simulink model "tqdtqr_rebuild_V3"  (R2021b)
settings: Solver=VariableStepAuto  StartTime=0.0  StopTime=10.0  RelTol=1e-3
undefined symbols (not defined in the file): ATQD_AfterTqMinGain_X_Deg, ATQD_APSCreepBaseTqD_X_kph, ATQD_APSCreepBaseTqD_Y_Deg, ATQD_APSCreepBaseTqR_X_kph, ATQD_APSCreepBaseTqR_Y_Deg, ATQD_APSCreepIterm_X_kph, ATQD_APSCreepIterm_Y_kph, ATQD_APSCreepPterm_X_kph, ATQD_APSCreepPterm_Y_kph, ATQD_APSDecReq_X_kph, ATQD_APSDecReq_Y_mps2, ATQD_APSDecReqCMD_X_kph, ATQD_APSDecReqTs_X_pct, ATQD_APSDecTimeGain_X_Deg, ATQD_APSDecTimeGain_Y_s, ATQD_APSReqLowSpd_X_Deg, ATQD_AutoHoldReleaseBPS_X_Deg, ATQD_AWDLoadTrqnsGain_X_kg, ATQD_AWDLoadTrqnsGain_Y_pct, ATQD_BOSEnBPSPosn_X_kph, ATQD_BOSMap_X_rpm, ATQD_BOSMap_Y_pct, ATQD_CreepBaseTqD_X_kph, ATQD_CreepBaseTqD_Y_Deg, ATQD_CreepBaseTqR_X_kph, ATQD_CreepBaseTqR_Y_Deg, ATQD_CreepBPSDisPosn_X_Deg, ATQD_CreepBPSDisPosnR_X_Deg, ATQD_CreepBPSEnPosn_X_Deg, ATQD_CreepBPSEnPosnR_X_Deg, ATQD_CreepDeltaTq_X_kph, ATQD_CreepIterm_X_kph, ATQD_CreepIterm_Y_kph, ATQD_CreepItermMaxLimit_X_pct, ATQD_CreepPreloadTime_X_kph, ATQD_CreepPreloadTq_X_kph, ATQD_CreepPreloadTq_Y_s, ATQD_CreepProtTq_X_Deg, ATQD_CreepPterm_X_kph, ATQD_CreepPterm_Y_kph, ATQD_CreepRrTqSpRat_X_rpm, ATQD_CreepRrTqSpRat_Y_Nm, ATQD_CreepTargetSpdD_X_pct, ATQD_CreepTargetSpdR_X_pct, ATQD_CreepUpLimitTq_X_rpm, ATQD_DecIneOPDHoldEnDelay_X_Deg, ATQD_DecIneOPDHoldEnDelay_Y_bar, ATQD_ECOTqMapD_X_rpm, ATQD_ECOTqMapD_Y_pct, ATQD_EMTqMapD_X_rpm, ATQD_EMTqMapD_Y_pct, ATQD_EOPDTqMapDCon_X_rpm, ATQD_EOPDTqMapDCon_Y_Deg, ATQD_EstInitVehWeight_X_c, ATQD_FAfterTqCMDGain_X_rpm, ATQD_FAfterTqCMDGain_Y_pct, ATQD_ForceLowSpd_X_Deg, ATQD_ForcePLimitSpd_X_Deg, ATQD_FrLossMAPLowV_X_rpm, ATQD_FrLossMAPLowV_Y_Nm ... (+949)
libraries: simulink x235, hcu_lib x208, tqr x63, tqd x6
(part 35 of 37)

== stateflow chart tqdtqr_rebuild_V3/Input_Convert/Signal function/SWC1 SWC2 status/SWC2_Subsystem/Speed Setting Mode/ACC Speed Setting ON/ACCSetSpd_2506 ==
  state MeterSpd
    state OFF_Error_Disable
      en:
      VTQD_ACCSetSpd_raw32 =  min(VTQD_ACCActiveMetSpdHi_raw32, VTQD_SpdLim4SetSpd_raw32);
      VTQD_ACCSetSpd_raw32 = max(VTQD_ACCActiveMetSpdLo_raw32, VTQD_ACCSetSpd_raw32);
      VTQD_ACCSavedSetSpd_raw32 = VTQD_ACCSetSpd_raw32;
      du:
      VTQD_ACCSetSpd_raw32 =  min(VTQD_ACCActiveMetSpdHi_raw32, VTQD_SpdLim4SetSpd_raw32);
      VTQD_ACCSetSpd_raw32 = max(VTQD_ACCActiveMetSpdLo_raw32, VTQD_ACCSetSpd_raw32);
      VTQD_ACCSavedSetSpd_raw32 = VTQD_ACCSetSpd_raw32;
    state Terminal
      %Do Nothing
    state Standby
      en:
      VTQD_ACCSetSpd_raw32 =  min(VTQD_ACCActiveMetSpdHi_raw32, VTQD_SpdLim4SetSpd_raw32);
      VTQD_ACCSetSpd_raw32 = max(VTQD_ACCActiveMetSpdLo_raw32, VTQD_ACCSetSpd_raw32);
      VTQD_ACCSavedSetSpd_raw32 = VTQD_ACCSetSpd_raw32;
      du:
      VTQD_ACCSetSpd_raw32 =  min(VTQD_ACCActiveMetSpdHi_raw32, VTQD_SpdLim4SetSpd_raw32);
      VTQD_ACCSetSpd_raw32 = max(VTQD_ACCActiveMetSpdLo_raw32, VTQD_ACCSetSpd_raw32);
      VTQD_ACCSavedSetSpd_raw32 = VTQD_ACCSetSpd_raw32;
    state Active_Override_ShutOff
      (default) -> (junction 749) : {VTQD_HoldResDet_flg = FALSE;
          |  VTQD_ACCSavedSetSpd_raw32 = VTQD_LastSetSpd_kph;
          |  VTQD_ACCSetSpd_raw32 = VTQD_ACCSavedSetSpd_raw32}
      MeterSpd.Active_Override_ShutOff -> (junction 830) [order 1]
      (junction 830) -> (junction 834) [order 1] : [VTQD_DistanceUnit_flg == VINP_Distanceunit_flg || VTQD_ACCSavedSetSpd_raw32 <= ONE_FLOAT]
      (junction 834) -> (junction 749) : {VTQD_ACCSetSpd_raw32 = min(VTQD_ACCActiveMetSpdHi_raw32, VTQD_ACCSavedSetSpd_raw32);
          |  VTQD_ACCSavedSetSpd_raw32 = VTQD_ACCSetSpd_raw32;}
      (junction 749) -> (junction 1142) [order 1] : [VINP_ADASACCSta_enum == ENUM_ADASACCSTA_ACTIVE]
      (junction 1142) -> (junction 1148) [order 1] : [(VTQD_SWC2ScrollUpSta_flg ||...
          |   VTQD_SWC2ScrollDownSta_flg ||...
          |   VTQD_SWC2ScrollUpSta_enum == ENUM_SWCBOTTONPRESS_SHORTPRESS ||...
          |   VTQD_SWC2ScrollDownSta_enum == ENUM_SWCBOTTONPRESS_SHORTPRESS) &&...
          |  VTQD_HoldResDet_flg]
          | %add20250114
      (junction 830) -> (junction 832) [order 2]
      (junction 837) -> (junction 834)
      (junction 749) -> (junction 798) [order 2]
      (junction 1142) -> (junction 1144) [order 2] : {VTQD_HoldResDet_flg = FALSE}
          | %add20250114
      (junction 1148) -> (junction 1146) : {VTQD_HoldResDet_flg = TRUE}
          | %add20250114
      (junction 832) -> (junction 819) [order 1] : [VINP_Distanceunit_flg]
      (junction 832) -> (junction 833) [order 2] : {VTQD_ACCSavedSetSpd_raw32 = (VTQD_ACCSavedSetSpd_raw32 * MPH2KPH)}
      (junction 819) -> (junction 827) : {VTQD_ACCSavedSetSpd_raw32 = (VTQD_ACCSavedSetSpd_raw32 * KPH2MPH)}
      (junction 1144) -> (junction 1146)
      (junction 1146) -> (junction 751)
      (junction 751) -> (junction 757) [order 1] : [VTQD_Set2MeterSpd_flg ||...
          |  VTQD_SetRoadSpdLim_flg]
      (junction 757) -> (junction 1115) [order 1] : [VTQD_Set2MeterSpd_flg]
      (junction 751) -> (junction 762) [order 2]
      (junction 757) -> (junction 759) [order 2] : {VTQD_ACCSetSpd_raw32 =  min(VTQD_ACCActiveMetSpdHi_raw32, VTQD_SpdLim4SetSpd_raw32);
          |  VTQD_ACCSetSpd_raw32 = max(VTQD_ACCActiveMetSpdLo_raw32, VTQD_ACCSetSpd_raw32);
          |  VTQD_ACCSavedSetSpd_raw32 = VTQD_ACCSetSpd_raw32;
          |  VTQD_DistanceUnit_flg = VINP_Distanceunit_flg;}
      (junction 1115) -> (junction 1114) : {VTQD_ACCSetSpd_raw32 =  min(VTQD_ACCActiveMetSpdHi_raw32, VVMC_MeterIndSpeed_raw32);
          |  VTQD_ACCSetSpd_raw32 = max(VTQD_ACCActiveMetSpdLo_raw32, VTQD_ACCSetSpd_raw32);
          |  VTQD_ACCSavedSetSpd_raw32 = VTQD_ACCSetSpd_raw32;
          |  VTQD_DistanceUnit_flg = VINP_Distanceunit_flg;}
      (junction 827) -> (junction 816) [order 1] : [VTQD_ACCSavedSetSpd_raw32 < KTQD_ACCActiveMetSpdLoMPH_mph]
      (junction 833) -> (junction 817) [order 1] : [VTQD_ACCSavedSetSpd_raw32 < KTQD_ACCActiveMetSpdLo_kph]
      (junction 816) -> (junction 820) : {VTQD_ACCSavedSetSpd_raw32 = KTQD_ACCActiveMetSpdLoMPH_mph}
      (junction 833) -> (junction 828) [order 2]
      (junction 817) -> (junction 815) : {VTQD_ACCSavedSetSpd_raw32 = KTQD_ACCActiveMetSpdLo_kph}
      (junction 827) -> (junction 818) [order 2]
      (junction 820) -> (junction 818)
      (junction 815) -> (junction 828)
      (junction 818) -> (junction 826)
      (junction 828) -> (junction 821)
      (junction 762) -> (junction 766) [order 1] : [(VTQD_SWC2ScrollUpSta_enum == ENUM_SWCBOTTONPRESS_SHORTPRESS ||...
          |   VTQD_SWC2ScrollDownSta_enum == ENUM_SWCBOTTONPRESS_SHORTPRESS) &&...
          |  !VVMC_LVDAACCStatusInformation_flg && !VTQD_HoldResDet_flg]
          | %add20250114
      (junction 766) -> (junction 771) [order 1] : [VTQD_SWC2ScrollUpSta_enum == ENUM_SWCBOTTONPRESS_SHORTPRESS]
      (junction 821) -> (junction 829) [order 1] : [VTQD_ACCSavedSetSpd_raw32 > KTQD_ACCActiveMetSpdHi_kph]
      (junction 826) -> (junction 822) [order 1] : [VTQD_ACCSavedSetSpd_raw32 > KTQD_ACCActiveMetSpdHiMPH_mph]
      (junction 762) -> (junction 792) [order 2]
      (junction 766) -> (junction 779) [order 2] : {VTQD_ACCSetSpd_raw32 =  min(VTQD_ACCActiveMetSpdHi_raw32, VTQD_ACCSavedSetSpd_raw32 - ONE_FLOAT);
          |  VTQD_ACCSetSpd_raw32 = max(VTQD_ACCActiveMetSpdLo_raw32, VTQD_ACCSetSpd_raw32);
          |  VTQD_ACCSavedSetSpd_raw32 = VTQD_ACCSetSpd_raw32;
          |  VTQD_DistanceUnit_flg = VINP_Distanceunit_flg;}
      (junction 771) -> (junction 774) : {VTQD_ACCSetSpd_raw32 =  min(VTQD_ACCActiveMetSpdHi_raw32, VTQD_ACCSavedSetSpd_raw32 + ONE_FLOAT);
          |  VTQD_ACCSetSpd_raw32 = max(VTQD_ACCActiveMetSpdLo_raw32, VTQD_ACCSetSpd_raw32);
          |  VTQD_ACCSavedSetSpd_raw32 = VTQD_ACCSetSpd_raw32;
          |  VTQD_DistanceUnit_flg = VINP_Distanceunit_flg;}
      (junction 821) -> (junction 823) [order 2]
      (junction 829) -> (junction 831) : {VTQD_ACCSavedSetSpd_raw32 = KTQD_ACCActiveMetSpdHi_kph}
      (junction 826) -> (junction 835) [order 2]
      (junction 822) -> (junction 824) : {VTQD_ACCSavedSetSpd_raw32 = KTQD_ACCActiveMetSpdHiMPH_mph}
      (junction 831) -> (junction 823)
      (junction 824) -> (junction 835)
      (junction 823) -> (junction 825)
      (junction 835) -> (junction 836)
      (junction 825) -> (junction 836)
      (junction 836) -> (junction 837)
      (junction 792) -> (junction 785) [order 1] : [(VTQD_SWC2ScrollUpSta_enum == ENUM_SWCBOTTONPRESS_LONGPRESS ||...
          |   VTQD_SWC2ScrollDownSta_enum == ENUM_SWCBOTTONPRESS_LONGPRESS) &&...
          |  !VVMC_LVDAACCStatusInformation_flg && !VTQD_HoldResDet_flg]
          | %add20250114
      (junction 785) -> (junction 790) [order 1] : [VTQD_SWC2ScrollUpSta_enum == ENUM_SWCBOTTONPRESS_LONGPRESS]
      (junction 792) -> (junction 1131) [order 2]
      (junction 785) -> (junction 793) [order 2] : {VTQD_ACCSetSpd_raw32 = max(VTQD_ACCActiveMetSpdLo_raw32, ceil(VTQD_ACCSavedSetSpd_raw32 / VTQD_SetSpdDeltaLong_raw32 - ONE_FLOAT) * VTQD_SetSpdDeltaLong_raw32);
          |  VTQD_ACCSetSpd_raw32 = min (VTQD_ACCActiveMetSpdHi_raw32, VTQD_ACCSetSpd_raw32);
          |  VTQD_ACCSavedSetSpd_raw32 = VTQD_ACCSetSpd_raw32;
          |  VTQD_DistanceUnit_flg = VINP_Distanceunit_flg;}
      (junction 790) -> (junction 783) : {VTQD_ACCSetSpd_raw32 = min(VTQD_ACCActiveMetSpdHi_raw32, floor(VTQD_ACCSavedSetSpd_raw32 / VTQD_SetSpdDeltaLong_raw32 + ONE_FLOAT) * VTQD_SetSpdDeltaLong_raw32);
          |  VTQD_ACCSetSpd_raw32 = max (VTQD_ACCActiveMetSpdLo_raw32, VTQD_ACCSetSpd_raw32);
          |  VTQD_ACCSavedSetSpd_raw32 = VTQD_ACCSetSpd_raw32;
          |  VTQD_DistanceUnit_flg = VINP_Distanceunit_flg;}
      (junction 1131) -> (junction 1133) [order 1] : [(VTQD_SWC2ScrollUpSta_flg ||...
          |   VTQD_SWC2ScrollDownSta_flg) &&...
          |  VVMC_LVDAACCStatusInformation_flg]
          | %add20250114
      (junction 1131) -> (junction 1137) [order 2]
      (junction 1133) -> (junction 1134) : {VTQD_HoldResDet_flg = TRUE}
          | %add20250114
      (junction 1134) -> (junction 1137)
      (junction 1137) -> (junction 1265) : {VTQD_ACCSetSpd_raw32 = VTQD_ACCSavedSetSpd_raw32;
          |  VTQD_ACCSavedSetSpd_raw32 = VTQD_ACCSetSpd_raw32;
          |  VTQD_DistanceUnit_flg = VINP_Distanceunit_flg;}
      (junction 798) -> (junction 1240) [order 1] : [VINP_ADASACCSta_enum == ENUM_ADASACCSTA_OVERRIDE]
      (junction 1240) -> (junction 1235) [order 1] : [KTQD_ACCOVRDSpdAdj_flg &&...
          | (VTQD_Set2MeterSpd_flg ||...
          |  VTQD_SetRoadSpdLim_flg)]
      (junction 1235) -> (junction 1247) [order 1] : [VTQD_Set2MeterSpd_flg]
      (junction 798) -> (junction 807) [order 2] : {VTQD_ACCSetSpd_raw32 = VTQD_ACCSavedSetSpd_raw32;
          |  VTQD_ACCSavedSetSpd_raw32 = VTQD_ACCSetSpd_raw32;
          |  VTQD_DistanceUnit_flg = VINP_Distanceunit_flg;}
      (junction 1240) -> (junction 1236) [order 2]
      (junction 1235) -> (junction 1244) [order 2] : {VTQD_ACCSetSpd_raw32 =  min(VTQD_ACCActiveMetSpdHi_raw32, VTQD_SpdLim4SetSpd_raw32);
          |  VTQD_ACCSetSpd_raw32 = max(VTQD_ACCActiveMetSpdLo_raw32, VTQD_ACCSetSpd_raw32);
          |  VTQD_ACCSavedSetSpd_raw32 = VTQD_ACCSetSpd_raw32;
          |  VTQD_DistanceUnit_flg = VINP_Distanceunit_flg;}
      (junction 1247) -> (junction 1241) : {VTQD_ACCSetSpd_raw32 =  min(VTQD_ACCActiveMetSpdHi_raw32, VVMC_MeterIndSpeed_raw32);
          |  VTQD_ACCSetSpd_raw32 = max(VTQD_ACCActiveMetSpdLo_raw32, VTQD_ACCSetSpd_raw32);
          |  VTQD_ACCSavedSetSpd_raw32 = VTQD_ACCSetSpd_raw32;
          |  VTQD_DistanceUnit_flg = VINP_Distanceunit_flg;}
      (junction 1236) -> (junction 1242) [order 1] : [(VTQD_SWC2ScrollUpSta_enum == ENUM_SWCBOTTONPRESS_SHORTPRESS ||...
          |   VTQD_SWC2ScrollDownSta_enum == ENUM_SWCBOTTONPRESS_SHORTPRESS)]
      (junction 1242) -> (junction 1238) [order 1] : [VTQD_SWC2ScrollUpSta_enum == ENUM_SWCBOTTONPRESS_SHORTPRESS]
      (junction 1236) -> (junction 1245) [order 2]
      (junction 1242) -> (junction 1248) [order 2] : {VTQD_ACCSetSpd_raw32 =  min(VTQD_ACCActiveMetSpdHi_raw32, VTQD_ACCSavedSetSpd_raw32 - ONE_FLOAT);
          |  VTQD_ACCSetSpd_raw32 = max(VTQD_ACCActiveMetSpdLo_raw32, VTQD_ACCSetSpd_raw32);
          |  VTQD_ACCSavedSetSpd_raw32 = VTQD_ACCSetSpd_raw32;
          |  VTQD_DistanceUnit_flg = VINP_Distanceunit_flg;}
      (junction 1238) -> (junction 1239) : {VTQD_ACCSetSpd_raw32 =  min(VTQD_ACCActiveMetSpdHi_raw32, VTQD_ACCSavedSetSpd_raw32 + ONE_FLOAT);
          |  VTQD_ACCSetSpd_raw32 = max(VTQD_ACCActiveMetSpdLo_raw32, VTQD_ACCSetSpd_raw32);
          |  VTQD_ACCSavedSetSpd_raw32 = VTQD_ACCSetSpd_raw32;
          |  VTQD_DistanceUnit_flg = VINP_Distanceunit_flg;}
      (junction 1245) -> (junction 1249) [order 1] : [(VTQD_SWC2ScrollUpSta_enum == ENUM_SWCBOTTONPRESS_LONGPRESS ||...
          |   VTQD_SWC2ScrollDownSta_enum == ENUM_SWCBOTTONPRESS_LONGPRESS)]
      (junction 1249) -> (junction 1243) [order 1] : [VTQD_SWC2ScrollUpSta_enum == ENUM_SWCBOTTONPRESS_LONGPRESS]
      (junction 1245) -> (junction 1234) [order 2] : {VTQD_ACCSetSpd_raw32 = VTQD_ACCSavedSetSpd_raw32;
          |  VTQD_ACCSavedSetSpd_raw32 = VTQD_ACCSetSpd_raw32;
          |  VTQD_DistanceUnit_flg = VINP_Distanceunit_flg;}
      (junction 1249) -> (junction 1246) [order 2] : {VTQD_ACCSetSpd_raw32 = max(VTQD_ACCActiveMetSpdLo_raw32, ceil(VTQD_ACCSavedSetSpd_raw32 / VTQD_SetSpdDeltaLong_raw32 - ONE_FLOAT) * VTQD_SetSpdDeltaLong_raw32);
          |  VTQD_ACCSetSpd_raw32 = min (VTQD_ACCActiveMetSpdHi_raw32, VTQD_ACCSetSpd_raw32);
          |  VTQD_ACCSavedSetSpd_raw32 = VTQD_ACCSetSpd_raw32;
          |  VTQD_DistanceUnit_flg = VINP_Distanceunit_flg;}
      (junction 1243) -> (junction 1237) : {VTQD_ACCSetSpd_raw32 = min(VTQD_ACCActiveMetSpdHi_raw32, floor(VTQD_ACCSavedSetSpd_raw32 / VTQD_SetSpdDeltaLong_raw32 + ONE_FLOAT) * VTQD_SetSpdDeltaLong_raw32);
          |  VTQD_ACCSetSpd_raw32 = max (VTQD_ACCActiveMetSpdLo_raw32, VTQD_ACCSetSpd_raw32);
          |  VTQD_ACCSavedSetSpd_raw32 = VTQD_ACCSetSpd_raw32;
          |  VTQD_DistanceUnit_flg = VINP_Distanceunit_flg;}
    (default) -> MeterSpd.OFF_Error_Disable [order 3]
    MeterSpd.Terminal -> MeterSpd.OFF_Error_Disable [order 2] : [VINP_ADASACCSta_enum ~= ENUM_ADASACCSTA_ACTIVE &&...
        |  VINP_ADASACCSta_enum ~= ENUM_ADASACCSTA_OVERRIDE &&...
        |  VINP_ADASACCSta_enum ~= ENUM_ADASACCSTA_SHUTOFF]
    MeterSpd.OFF_Error_Disable -> MeterSpd.Terminal [order 2] : [VINP_ADASACCSta_enum == ENUM_ADASACCSTA_ACTIVE ||...
        |  VINP_ADASACCSta_enum == ENUM_ADASACCSTA_OVERRIDE ||...
        |  VINP_ADASACCSta_enum == ENUM_ADASACCSTA_SHUTOFF]
    MeterSpd.Terminal -> MeterSpd.Active_Override_ShutOff [order 1] : [VINP_ADASACCSta_enum == ENUM_ADASACCSTA_ACTIVE ||...
        |  VINP_ADASACCSta_enum == ENUM_ADASACCSTA_OVERRIDE ||...
        |  VINP_ADASACCSta_enum == ENUM_ADASACCSTA_SHUTOFF]
    MeterSpd.Active_Override_ShutOff -> MeterSpd.Terminal [order 2] : [VINP_ADASACCSta_enum ~= ENUM_ADASACCSTA_ACTIVE &&...
        |  VINP_ADASACCSta_enum ~= ENUM_ADASACCSTA_OVERRIDE &&...
        |  VINP_ADASACCSta_enum ~= ENUM_ADASACCSTA_SHUTOFF]
    MeterSpd.OFF_Error_Disable -> MeterSpd.Standby [order 1] : [VINP_ADASACCSta_enum == ENUM_ADASACCSTA_STANDBY]
    MeterSpd.Standby -> MeterSpd.OFF_Error_Disable [order 2] : [VINP_ADASACCSta_enum ~= ENUM_ADASACCSTA_STANDBY]
    MeterSpd.Active_Override_ShutOff -> MeterSpd.Standby [order 1] : [VINP_ADASACCSta_enum == ENUM_ADASACCSTA_STANDBY]
    MeterSpd.Standby -> MeterSpd.Active_Override_ShutOff [order 1] : [VINP_ADASACCSta_enum == ENUM_ADASACCSTA_ACTIVE ||...
        |  VINP_ADASACCSta_enum == ENUM_ADASACCSTA_OVERRIDE ||...
        |  VINP_ADASACCSta_enum == ENUM_ADASACCSTA_SHUTOFF]
    (default) -> MeterSpd.Active_Override_ShutOff [order 2] : [VINP_ADASACCSta_enum == ENUM_ADASACCSTA_ACTIVE ||...
        |  VINP_ADASACCSta_enum == ENUM_ADASACCSTA_OVERRIDE ||...
        |  VINP_ADASACCSta_enum == ENUM_ADASACCSTA_SHUTOFF]
    (default) -> MeterSpd.Standby [order 1] : [VINP_ADASACCSta_enum == ENUM_ADASACCSTA_STANDBY]
  state RoadSpd
    state OFF_Error_Disable
      en:
      VTQD_ACCSetSpd_raw32 =  min(VTQD_ACCActiveMetSpdHi_raw32, VTQD_SpdLim4SetSpd_raw32);
      VTQD_ACCSetSpd_raw32 = max(VTQD_ACCActiveMetSpdLo_raw32, VTQD_ACCSetSpd_raw32);
      VTQD_ACCSavedSetSpd_raw32 = VTQD_ACCSetSpd_raw32;
      du:
      VTQD_ACCSetSpd_raw32 =  min(VTQD_ACCActiveMetSpdHi_raw32, VTQD_SpdLim4SetSpd_raw32);
      VTQD_ACCSetSpd_raw32 = max(VTQD_ACCActiveMetSpdLo_raw32, VTQD_ACCSetSpd_raw32);
      VTQD_ACCSavedSetSpd_raw32 = VTQD_ACCSetSpd_raw32;
    state Terminal
      %Do Nothing
    state Standby
      (default) -> (junction 987) : {VTQD_StandbyDisRoadSpd_flg = FALSE;}
      RoadSpd.Standby -> (junction 1029) [order 1]
      (junction 1029) -> (junction 1030) [order 1] : [VTQD_DistanceUnit_flg == VINP_Distanceunit_flg || VTQD_ACCSavedSetSpd_raw32 <= ONE_FLOAT]
      (junction 1030) -> (junction 987) : {VTQD_ACCSetSpd_raw32 = min(VTQD_ACCActiveMetSpdHi_raw32, VTQD_ACCSavedSetSpd_raw32);
          |  VTQD_ACCSavedSetSpd_raw32 = VTQD_ACCSetSpd_raw32;}
      (junction 987) -> (junction 1102) [order 1] : [VTQD_RoadSpdActive2Standby_flg &&...
          | (VTQD_StandbyDisRoadSpd_flg || !VTQD_ADASSLIFSpdLimDet_flg)]
      (junction 1029) -> (junction 1031) [order 2]
      (junction 1048) -> (junction 1030)
      (junction 987) -> (junction 1104) [order 2]
      (junction 1102) -> (junction 999)
      (junction 1031) -> (junction 1032) [order 1] : [VINP_Distanceunit_flg]
      (junction 1031) -> (junction 1034) [order 2] : {VTQD_ACCSavedSetSpd_raw32 = (VTQD_ACCSavedSetSpd_raw32 * MPH2KPH)}
      (junction 1032) -> (junction 1028) : {VTQD_ACCSavedSetSpd_raw32 = (VTQD_ACCSavedSetSpd_raw32 * KPH2MPH)}
      (junction 1104) -> (junction 999) [order 1] : [VTQD_SWC2ScrollUpSta_enum ~= ENUM_SWCBOTTONPRESS_NOPRESS ||...
          |  VTQD_SWC2ScrollDownSta_enum ~= ENUM_SWCBOTTONPRESS_NOPRESS ||...
          |  VTQD_StandbyDisRoadSpd_flg]
      (junction 999) -> (junction 1000) [order 1] : [VTQD_SWC2ScrollUpSta_enum == ENUM_SWCBOTTONPRESS_SHORTPRESS ||...
          |  VTQD_SWC2ScrollDownSta_enum == ENUM_SWCBOTTONPRESS_SHORTPRESS]
      (junction 1000) -> (junction 1001) [order 1] : [VTQD_SWC2ScrollUpSta_enum == ENUM_SWCBOTTONPRESS_SHORTPRESS]
      (junction 1104) -> (junction 991) [order 2] : {VTQD_ACCSetSpd_raw32 =  min(VTQD_ACCActiveMetSpdHi_raw32, VTQD_SpdLim4SetSpd_raw32);
          |  VTQD_ACCSetSpd_raw32 = max(VTQD_ACCActiveMetSpdLo_raw32, VTQD_ACCSetSpd_raw32);
          |  VTQD_ACCSavedSetSpd_raw32 = VTQD_ACCSetSpd_raw32;
          |  VTQD_DistanceUnit_flg = VINP_Distanceunit_flg;
          |  VTQD_RoadSpdActive2Standby_flg = FALSE;}
      (junction 999) -> (junction 1007) [order 2]
      (junction 1000) -> (junction 1005) [order 2] : {VTQD_ACCSetSpd_raw32 =  min(VTQD_ACCActiveMetSpdHi_raw32, VTQD_ACCSavedSetSpd_raw32 - ONE_FLOAT);
          |  VTQD_ACCSetSpd_raw32 = max(VTQD_ACCActiveMetSpdLo_raw32, VTQD_ACCSetSpd_raw32);
          |  VTQD_ACCSavedSetSpd_raw32 = VTQD_ACCSetSpd_raw32;
          |  VTQD_DistanceUnit_flg = VINP_Distanceunit_flg;
          |  VTQD_StandbyDisRoadSpd_flg = TRUE;}
      (junction 1001) -> (junction 1006) : {VTQD_ACCSetSpd_raw32 =  min(VTQD_ACCActiveMetSpdHi_raw32, VTQD_ACCSavedSetSpd_raw32 + ONE_FLOAT);
          |  VTQD_ACCSetSpd_raw32 = max(VTQD_ACCActiveMetSpdLo_raw32, VTQD_ACCSetSpd_raw32);
          |  VTQD_ACCSavedSetSpd_raw32 = VTQD_ACCSetSpd_raw32;
          |  VTQD_DistanceUnit_flg = VINP_Distanceunit_flg;
          |  VTQD_StandbyDisRoadSpd_flg = TRUE;}
      (junction 1028) -> (junction 1033) [order 1] : [VTQD_ACCSavedSetSpd_raw32 < KTQD_ACCActiveMetSpdLoMPH_mph]
      (junction 1034) -> (junction 1035) [order 1] : [VTQD_ACCSavedSetSpd_raw32 < KTQD_ACCActiveMetSpdLo_kph]
      (junction 1033) -> (junction 1043) : {VTQD_ACCSavedSetSpd_raw32 = KTQD_ACCActiveMetSpdLoMPH_mph}
      (junction 1034) -> (junction 1038) [order 2]
      (junction 1035) -> (junction 1039) : {VTQD_ACCSavedSetSpd_raw32 = KTQD_ACCActiveMetSpdLo_kph}
      (junction 1028) -> (junction 1045) [order 2]
      (junction 1043) -> (junction 1045)
      (junction 1039) -> (junction 1038)
      (junction 1045) -> (junction 1042)
      (junction 1038) -> (junction 1040)
      (junction 1040) -> (junction 1041) [order 1] : [VTQD_ACCSavedSetSpd_raw32 > KTQD_ACCActiveMetSpdHi_kph]
      (junction 1042) -> (junction 1044) [order 1] : [VTQD_ACCSavedSetSpd_raw32 > KTQD_ACCActiveMetSpdHiMPH_mph]
      (junction 1040) -> (junction 1053) [order 2]
      (junction 1041) -> (junction 1049) : {VTQD_ACCSavedSetSpd_raw32 = KTQD_ACCActiveMetSpdHi_kph}
      (junction 1042) -> (junction 1054) [order 2]
      (junction 1044) -> (junction 1047) : {VTQD_ACCSavedSetSpd_raw32 = KTQD_ACCActiveMetSpdHiMPH_mph}
      (junction 1007) -> (junction 1011) [order 1] : [VTQD_SWC2ScrollUpSta_enum == ENUM_SWCBOTTONPRESS_LONGPRESS ||...
          |  VTQD_SWC2ScrollDownSta_enum == ENUM_SWCBOTTONPRESS_LONGPRESS]
      (junction 1011) -> (junction 1009) [order 1] : [VTQD_SWC2ScrollUpSta_enum == ENUM_SWCBOTTONPRESS_LONGPRESS]
      (junction 1007) -> (junction 1012) [order 2]
      (junction 1011) -> (junction 1010) [order 2] : {VTQD_ACCSetSpd_raw32 = max(VTQD_ACCActiveMetSpdLo_raw32, ceil(VTQD_ACCSavedSetSpd_raw32 / VTQD_SetSpdDeltaLong_raw32 - ONE_FLOAT) * VTQD_SetSpdDeltaLong_raw32);
          |  VTQD_ACCSetSpd_raw32 = min (VTQD_ACCActiveMetSpdHi_raw32, VTQD_ACCSetSpd_raw32);
          |  VTQD_ACCSavedSetSpd_raw32 = VTQD_ACCSetSpd_raw32;
          |  VTQD_DistanceUnit_flg = VINP_Distanceunit_flg;
          |  VTQD_StandbyDisRoadSpd_flg = TRUE;}
      (junction 1009) -> (junction 1008) : {VTQD_ACCSetSpd_raw32 = min(VTQD_ACCActiveMetSpdHi_raw32, floor(VTQD_ACCSavedSetSpd_raw32 / VTQD_SetSpdDeltaLong_raw32 + ONE_FLOAT) * VTQD_SetSpdDeltaLong_raw32);
          |  VTQD_ACCSetSpd_raw32 = max (VTQD_ACCActiveMetSpdLo_raw32, VTQD_ACCSetSpd_raw32);
          |  VTQD_ACCSavedSetSpd_raw32 = VTQD_ACCSetSpd_raw32;
          |  VTQD_DistanceUnit_flg = VINP_Distanceunit_flg;
          |  VTQD_StandbyDisRoadSpd_flg = TRUE;}
      (junction 1049) -> (junction 1053)
      (junction 1047) -> (junction 1054)
      (junction 1053) -> (junction 1046)
      (junction 1054) -> (junction 1050)
      (junction 1046) -> (junction 1050)
      (junction 1050) -> (junction 1048)
      (junction 1012) -> (junction 1023) [order 1] : [VTQD_LScrollPressShort_flg &&...
          |  VTQD_ADASSLIFSpdLimDet_flg]
      (junction 1023) -> (junction 1026) : {VTQD_ACCSetSpd_raw32 =  min(VTQD_ACCActiveMetSpdHi_raw32, VTQD_SpdLim4SetSpd_raw32);
          |  VTQD_ACCSetSpd_raw32 = max(VTQD_ACCActiveMetSpdLo_raw32, VTQD_ACCSetSpd_raw32);
          |  VTQD_ACCSavedSetSpd_raw32 = VTQD_ACCSetSpd_raw32;
          |  VTQD_DistanceUnit_flg = VINP_Distanceunit_flg;
          |  VTQD_StandbyDisRoadSpd_flg = FALSE;
          |  VTQD_RoadSpdActive2Standby_flg = FALSE;}
      (junction 1012) -> (junction 1022) [order 2] : {VTQD_ACCSetSpd_raw32 =  VTQD_ACCSavedSetSpd_raw32;
          |  VTQD_ACCSavedSetSpd_raw32 = VTQD_ACCSetSpd_raw32;
          |  VTQD_DistanceUnit_flg = VINP_Distanceunit_flg;}
    state Active_Override_ShutOff
      (default) -> (junction 883) : {VTQD_HoldResDet_flg = FALSE;
          |  VTQD_ACCSavedSetSpd_raw32 = VTQD_LastSetSpd_kph;
          |  VTQD_ACCSetSpd_raw32 = VTQD_ACCSavedSetSpd_raw32}
      RoadSpd.Active_Override_ShutOff -> (junction 881) [order 1]
      (junction 881) -> (junction 882) [order 1] : [VTQD_DistanceUnit_flg == VINP_Distanceunit_flg || VTQD_ACCSavedSetSpd_raw32 <= ONE_FLOAT]
      (junction 882) -> (junction 883) : {VTQD_ACCSetSpd_raw32 = min(VTQD_ACCActiveMetSpdHi_raw32, VTQD_ACCSavedSetSpd_raw32);
          |  VTQD_ACCSavedSetSpd_raw32 = VTQD_ACCSetSpd_raw32;}
      (junction 883) -> (junction 1190) [order 1] : [VINP_ADASACCSta_enum == ENUM_ADASACCSTA_ACTIVE]
      (junction 1190) -> (junction 1197) [order 1] : [(VTQD_SWC2ScrollUpSta_flg ||...
          |   VTQD_SWC2ScrollDownSta_flg ||...
          |   VTQD_SWC2ScrollUpSta_enum == ENUM_SWCBOTTONPRESS_SHORTPRESS ||...
          |   VTQD_SWC2ScrollDownSta_enum == ENUM_SWCBOTTONPRESS_SHORTPRESS) &&...
          |  VTQD_HoldResDet_flg]
          | %add20250114
      (junction 881) -> (junction 886) [order 2]
      (junction 915) -> (junction 882)
      (junction 883) -> (junction 919) [order 2]
      (junction 1190) -> (junction 1193) [order 2] : {VTQD_HoldResDet_flg = FALSE}
          | %add20250114
      (junction 1197) -> (junction 1195) : {VTQD_HoldResDet_flg = TRUE}
          | %add20250114
      (junction 886) -> (junction 887) [order 1] : [VINP_Distanceunit_flg]
      (junction 886) -> (junction 893) [order 2] : {VTQD_ACCSavedSetSpd_raw32 = (VTQD_ACCSavedSetSpd_raw32 * MPH2KPH)}
      (junction 887) -> (junction 895) : {VTQD_ACCSavedSetSpd_raw32 = (VTQD_ACCSavedSetSpd_raw32 * KPH2MPH)}
      (junction 1193) -> (junction 1195)
      (junction 1195) -> (junction 884)
      (junction 884) -> (junction 885) [order 1] : [VTQD_Set2MeterSpd_flg ||...
          |  VTQD_SetRoadSpdLim_flg]
      (junction 885) -> (junction 1124) [order 1] : [VTQD_Set2MeterSpd_flg]
      (junction 884) -> (junction 889) [order 2]
      (junction 885) -> (junction 888) [order 2] : {VTQD_ACCSetSpd_raw32 =  min(VTQD_ACCActiveMetSpdHi_raw32, VTQD_SpdLim4SetSpd_raw32);
          |  VTQD_ACCSetSpd_raw32 = max(VTQD_ACCActiveMetSpdLo_raw32, VTQD_ACCSetSpd_raw32);
          |  VTQD_ACCSavedSetSpd_raw32 = VTQD_ACCSetSpd_raw32;
          |  VTQD_DistanceUnit_flg = VINP_Distanceunit_flg;}
      (junction 1124) -> (junction 1123) : {VTQD_ACCSetSpd_raw32 =  min(VTQD_ACCActiveMetSpdHi_raw32, VVMC_MeterIndSpeed_raw32);
          |  VTQD_ACCSetSpd_raw32 = max(VTQD_ACCActiveMetSpdLo_raw32, VTQD_ACCSetSpd_raw32);
          |  VTQD_ACCSavedSetSpd_raw32 = VTQD_ACCSetSpd_raw32;
          |  VTQD_DistanceUnit_flg = VINP_Distanceunit_flg;}
      (junction 895) -> (junction 892) [order 1] : [VTQD_ACCSavedSetSpd_raw32 < KTQD_ACCActiveMetSpdLoMPH_mph]
      (junction 893) -> (junction 894) [order 1] : [VTQD_ACCSavedSetSpd_raw32 < KTQD_ACCActiveMetSpdLo_kph]
      (junction 892) -> (junction 897) : {VTQD_ACCSavedSetSpd_raw32 = KTQD_ACCActiveMetSpdLoMPH_mph}
      (junction 893) -> (junction 898) [order 2]
      (junction 894) -> (junction 899) : {VTQD_ACCSavedSetSpd_raw32 = KTQD_ACCActiveMetSpdLo_kph}
      (junction 895) -> (junction 896) [order 2]
      (junction 897) -> (junction 896)
      (junction 899) -> (junction 898)
      (junction 896) -> (junction 902)
      (junction 898) -> (junction 900)
      (junction 889) -> (junction 890) [order 1] : [(VTQD_SWC2ScrollUpSta_enum == ENUM_SWCBOTTONPRESS_SHORTPRESS ||...
          |   VTQD_SWC2ScrollDownSta_enum == ENUM_SWCBOTTONPRESS_SHORTPRESS) &&...
          |  !VVMC_LVDAACCStatusInformation_flg && !VTQD_HoldResDet_flg]
          | %add20250114
      (junction 890) -> (junction 891) [order 1] : [VTQD_SWC2ScrollUpSta_enum == ENUM_SWCBOTTONPRESS_SHORTPRESS]
      (junction 900) -> (junction 901) [order 1] : [VTQD_ACCSavedSetSpd_raw32 > KTQD_ACCActiveMetSpdHi_kph]
      (junction 902) -> (junction 903) [order 1] : [VTQD_ACCSavedSetSpd_raw32 > KTQD_ACCActiveMetSpdHiMPH_mph]
      (junction 889) -> (junction 906) [order 2]
      (junction 890) -> (junction 904) [order 2] : {VTQD_ACCSetSpd_raw32 =  min(VTQD_ACCActiveMetSpdHi_raw32, VTQD_ACCSavedSetSpd_raw32 - ONE_FLOAT);
          |  VTQD_ACCSetSpd_raw32 = max(VTQD_ACCActiveMetSpdLo_raw32, VTQD_ACCSetSpd_raw32);
          |  VTQD_ACCSavedSetSpd_raw32 = VTQD_ACCSetSpd_raw32;
          |  VTQD_DistanceUnit_flg = VINP_Distanceunit_flg;}
      (junction 891) -> (junction 905) : {VTQD_ACCSetSpd_raw32 =  min(VTQD_ACCActiveMetSpdHi_raw32, VTQD_ACCSavedSetSpd_raw32 + ONE_FLOAT);
          |  VTQD_ACCSetSpd_raw32 = max(VTQD_ACCActiveMetSpdLo_raw32, VTQD_ACCSetSpd_raw32);
          |  VTQD_ACCSavedSetSpd_raw32 = VTQD_ACCSetSpd_raw32;
          |  VTQD_DistanceUnit_flg = VINP_Distanceunit_flg;}
      (junction 900) -> (junction 909) [order 2]
      (junction 901) -> (junction 910) : {VTQD_ACCSavedSetSpd_raw32 = KTQD_ACCActiveMetSpdHi_kph}
      (junction 902) -> (junction 911) [order 2]
      (junction 903) -> (junction 912) : {VTQD_ACCSavedSetSpd_raw32 = KTQD_ACCActiveMetSpdHiMPH_mph}
      (junction 910) -> (junction 909)
      (junction 912) -> (junction 911)
      (junction 909) -> (junction 913)
      (junction 911) -> (junction 914)
      (junction 913) -> (junction 914)
      (junction 914) -> (junction 915)
      (junction 906) -> (junction 907) [order 1] : [(VTQD_SWC2ScrollUpSta_enum == ENUM_SWCBOTTONPRESS_LONGPRESS ||...
          |   VTQD_SWC2ScrollDownSta_enum == ENUM_SWCBOTTONPRESS_LONGPRESS) &&...
          |  !VVMC_LVDAACCStatusInformation_flg && !VTQD_HoldResDet_flg]
          | %add20250114
      (junction 907) -> (junction 908) [order 1] : [VTQD_SWC2ScrollUpSta_enum == ENUM_SWCBOTTONPRESS_LONGPRESS]
      (junction 906) -> (junction 1200) [order 2]
      (junction 907) -> (junction 917) [order 2] : {VTQD_ACCSetSpd_raw32 = max(VTQD_ACCActiveMetSpdLo_raw32, ceil(VTQD_ACCSavedSetSpd_raw32 / VTQD_SetSpdDeltaLong_raw32 - ONE_FLOAT) * VTQD_SetSpdDeltaLong_raw32);
          |  VTQD_ACCSetSpd_raw32 = min (VTQD_ACCActiveMetSpdHi_raw32, VTQD_ACCSetSpd_raw32);
          |  VTQD_ACCSavedSetSpd_raw32 = VTQD_ACCSetSpd_raw32;
          |  VTQD_DistanceUnit_flg = VINP_Distanceunit_flg;}
      (junction 908) -> (junction 918) : {VTQD_ACCSetSpd_raw32 = min(VTQD_ACCActiveMetSpdHi_raw32, floor(VTQD_ACCSavedSetSpd_raw32 / VTQD_SetSpdDeltaLong_raw32 + ONE_FLOAT) * VTQD_SetSpdDeltaLong_raw32);
          |  VTQD_ACCSetSpd_raw32 = max (VTQD_ACCActiveMetSpdLo_raw32, VTQD_ACCSetSpd_raw32);
          |  VTQD_ACCSavedSetSpd_raw32 = VTQD_ACCSetSpd_raw32;
          |  VTQD_DistanceUnit_flg = VINP_Distanceunit_flg;}
      (junction 1200) -> (junction 1209) [order 1] : [(VTQD_SWC2ScrollUpSta_flg ||...
          |   VTQD_SWC2ScrollDownSta_flg) &&...
          |  VVMC_LVDAACCStatusInformation_flg]
          | %add20250114
      (junction 1200) -> (junction 1202) [order 2]
      (junction 1209) -> (junction 1207) : {VTQD_HoldResDet_flg = TRUE}
          | %add20250114
      (junction 1207) -> (junction 1202)
      (junction 1202) -> (junction 1204) : {VTQD_ACCSetSpd_raw32 = VTQD_ACCSavedSetSpd_raw32;
          |  VTQD_ACCSavedSetSpd_raw32 = VTQD_ACCSetSpd_raw32;
          |  VTQD_DistanceUnit_flg = VINP_Distanceunit_flg;}
      (junction 919) -> (junction 1278) [order 1] : [VINP_ADASACCSta_enum == ENUM_ADASACCSTA_OVERRIDE]
      (junction 1278) -> (junction 1266) [order 1] : [KTQD_ACCOVRDSpdAdj_flg &&...
          | (VTQD_Set2MeterSpd_flg ||...
          |  VTQD_SetRoadSpdLim_flg)]
      (junction 1266) -> (junction 1277) [order 1] : [VTQD_Set2MeterSpd_flg]
      (junction 919) -> (junction 924) [order 2] : {VTQD_ACCSetSpd_raw32 = VTQD_ACCSavedSetSpd_raw32;
          |  VTQD_ACCSavedSetSpd_raw32 = VTQD_ACCSetSpd_raw32;
          |  VTQD_DistanceUnit_flg = VINP_Distanceunit_flg;}
      (junction 1278) -> (junction 1268) [order 2]
      (junction 1266) -> (junction 1272) [order 2] : {VTQD_ACCSetSpd_raw32 =  min(VTQD_ACCActiveMetSpdHi_raw32, VTQD_SpdLim4SetSpd_raw32);
          |  VTQD_ACCSetSpd_raw32 = max(VTQD_ACCActiveMetSpdLo_raw32, VTQD_ACCSetSpd_raw32);
          |  VTQD_ACCSavedSetSpd_raw32 = VTQD_ACCSetSpd_raw32;
          |  VTQD_DistanceUnit_flg = VINP_Distanceunit_flg;}
      (junction 1277) -> (junction 1269) : {VTQD_ACCSetSpd_raw32 =  min(VTQD_ACCActiveMetSpdHi_raw32, VVMC_MeterIndSpeed_raw32);
          |  VTQD_ACCSetSpd_raw32 = max(VTQD_ACCActiveMetSpdLo_raw32, VTQD_ACCSetSpd_raw32);
          |  VTQD_ACCSavedSetSpd_raw32 = VTQD_ACCSetSpd_raw32;
          |  VTQD_DistanceUnit_flg = VINP_Distanceunit_flg;}
      (junction 1268) -> (junction 1280) [order 1] : [(VTQD_SWC2ScrollUpSta_enum == ENUM_SWCBOTTONPRESS_SHORTPRESS ||...
          |   VTQD_SWC2ScrollDownSta_enum == ENUM_SWCBOTTONPRESS_SHORTPRESS)]
      (junction 1280) -> (junction 1270) [order 1] : [VTQD_SWC2ScrollUpSta_enum == ENUM_SWCBOTTONPRESS_SHORTPRESS]
      (junction 1268) -> (junction 1276) [order 2]
      (junction 1280) -> (junction 1279) [order 2] : {VTQD_ACCSetSpd_raw32 =  min(VTQD_ACCActiveMetSpdHi_raw32, VTQD_ACCSavedSetSpd_raw32 - ONE_FLOAT);
          |  VTQD_ACCSetSpd_raw32 = max(VTQD_ACCActiveMetSpdLo_raw32, VTQD_ACCSetSpd_raw32);
          |  VTQD_ACCSavedSetSpd_raw32 = VTQD_ACCSetSpd_raw32;
          |  VTQD_DistanceUnit_flg = VINP_Distanceunit_flg;}
      (junction 1270) -> (junction 1274) : {VTQD_ACCSetSpd_raw32 =  min(VTQD_ACCActiveMetSpdHi_raw32, VTQD_ACCSavedSetSpd_raw32 + ONE_FLOAT);
          |  VTQD_ACCSetSpd_raw32 = max(VTQD_ACCActiveMetSpdLo_raw32, VTQD_ACCSetSpd_raw32);
          |  VTQD_ACCSavedSetSpd_raw32 = VTQD_ACCSetSpd_raw32;
          |  VTQD_DistanceUnit_flg = VINP_Distanceunit_flg;}
      (junction 1276) -> (junction 1285) [order 1] : [(VTQD_SWC2ScrollUpSta_enum == ENUM_SWCBOTTONPRESS_LONGPRESS ||...
          |   VTQD_SWC2ScrollDownSta_enum == ENUM_SWCBOTTONPRESS_LONGPRESS)]
      (junction 1285) -> (junction 1271) [order 1] : [VTQD_SWC2ScrollUpSta_enum == ENUM_SWCBOTTONPRESS_LONGPRESS]
      (junction 1276) -> (junction 1267) [order 2] : {VTQD_ACCSetSpd_raw32 = VTQD_ACCSavedSetSpd_raw32;
          |  VTQD_ACCSavedSetSpd_raw32 = VTQD_ACCSetSpd_raw32;
          |  VTQD_DistanceUnit_flg = VINP_Distanceunit_flg;}
      (junction 1285) -> (junction 1275) [order 2] : {VTQD_ACCSetSpd_raw32 = max(VTQD_ACCActiveMetSpdLo_raw32, ceil(VTQD_ACCSavedSetSpd_raw32 / VTQD_SetSpdDeltaLong_raw32 - ONE_FLOAT) * VTQD_SetSpdDeltaLong_raw32);
          |  VTQD_ACCSetSpd_raw32 = min (VTQD_ACCActiveMetSpdHi_raw32, VTQD_ACCSetSpd_raw32);
          |  VTQD_ACCSavedSetSpd_raw32 = VTQD_ACCSetSpd_raw32;
          |  VTQD_DistanceUnit_flg = VINP_Distanceunit_flg;}
      (junction 1271) -> (junction 1273) : {VTQD_ACCSetSpd_raw32 = min(VTQD_ACCActiveMetSpdHi_raw32, floor(VTQD_ACCSavedSetSpd_raw32 / VTQD_SetSpdDeltaLong_raw32 + ONE_FLOAT) * VTQD_SetSpdDeltaLong_raw32);
          |  VTQD_ACCSetSpd_raw32 = max (VTQD_ACCActiveMetSpdLo_raw32, VTQD_ACCSetSpd_raw32);
          |  VTQD_ACCSavedSetSpd_raw32 = VTQD_ACCSetSpd_raw32;
          |  VTQD_DistanceUnit_flg = VINP_Distanceunit_flg;}
    (default) -> RoadSpd.OFF_Error_Disable [order 3]
    RoadSpd.Terminal -> RoadSpd.OFF_Error_Disable [order 2] : [VINP_ADASACCSta_enum ~= ENUM_ADASACCSTA_ACTIVE &&...
        |  VINP_ADASACCSta_enum ~= ENUM_ADASACCSTA_OVERRIDE &&...
        |  VINP_ADASACCSta_enum ~= ENUM_ADASACCSTA_SHUTOFF]
    RoadSpd.OFF_Error_Disable -> RoadSpd.Terminal [order 2] : [VINP_ADASACCSta_enum == ENUM_ADASACCSTA_ACTIVE ||...
        |  VINP_ADASACCSta_enum == ENUM_ADASACCSTA_OVERRIDE ||...
        |  VINP_ADASACCSta_enum == ENUM_ADASACCSTA_SHUTOFF]
        | {VTQD_RoadSpdActive2Standby_flg = FALSE;}
    RoadSpd.Terminal -> RoadSpd.Active_Override_ShutOff [order 1] : [VINP_ADASACCSta_enum == ENUM_ADASACCSTA_ACTIVE ||...
        |  VINP_ADASACCSta_enum == ENUM_ADASACCSTA_OVERRIDE ||...
        |  VINP_ADASACCSta_enum == ENUM_ADASACCSTA_SHUTOFF]
    RoadSpd.Active_Override_ShutOff -> RoadSpd.Terminal [order 2] : [VINP_ADASACCSta_enum ~= ENUM_ADASACCSTA_ACTIVE &&...
        |  VINP_ADASACCSta_enum ~= ENUM_ADASACCSTA_OVERRIDE &&...
        |  VINP_ADASACCSta_enum ~= ENUM_ADASACCSTA_SHUTOFF]
    RoadSpd.OFF_Error_Disable -> RoadSpd.Standby [order 1] : [VINP_ADASACCSta_enum == ENUM_ADASACCSTA_STANDBY]
    RoadSpd.Standby -> RoadSpd.OFF_Error_Disable [order 2] : [VINP_ADASACCSta_enum ~= ENUM_ADASACCSTA_STANDBY]
        | {VTQD_RoadSpdActive2Standby_flg = FALSE;}
    RoadSpd.Active_Override_ShutOff -> RoadSpd.Standby [order 1] : [VINP_ADASACCSta_enum == ENUM_ADASACCSTA_STANDBY]
        | {VTQD_RoadSpdActive2Standby_flg = TRUE;}
    RoadSpd.Standby -> RoadSpd.Active_Override_ShutOff [order 1] : [VINP_ADASACCSta_enum == ENUM_ADASACCSTA_ACTIVE ||...
        |  VINP_ADASACCSta_enum == ENUM_ADASACCSTA_OVERRIDE ||...
        |  VINP_ADASACCSta_enum == ENUM_ADASACCSTA_SHUTOFF]
        | {VTQD_RoadSpdActive2Standby_flg = FALSE;}
    (default) -> RoadSpd.Active_Override_ShutOff [order 2] : [VINP_ADASACCSta_enum == ENUM_ADASACCSTA_ACTIVE ||...
        |  VINP_ADASACCSta_enum == ENUM_ADASACCSTA_OVERRIDE ||...
        |  VINP_ADASACCSta_enum == ENUM_ADASACCSTA_SHUTOFF]
    (default) -> RoadSpd.Standby [order 1] : [VINP_ADASACCSta_enum == ENUM_ADASACCSTA_STANDBY]
  (default) -> MeterSpd : {VTQD_ACCSavedSetSpd_raw32 = ZERO_FLOAT;
      |  VTQD_RoadSpdActive2Standby_flg = FALSE;
      |  VTQD_StandbyDisRoadSpd_flg = FALSE}
  RoadSpd -> MeterSpd : [!VINP_IVIACCAdaptiveSta_flg]
  MeterSpd -> RoadSpd : [VINP_IVIACCAdaptiveSta_flg]
  data: VINP_ADASACCSta_enum input; ENUM_ADASACCSTA_SHUTOFF parameter; ENUM_ADASACCSTA_STANDBY parameter; ENUM_ADASACCSTA_OVERRIDE parameter; ENUM_ADASACCSTA_ACTIVE parameter; ZERO_FLOAT parameter; VTQD_ACCSetSpd_raw32 output single; VINP_IVIACCAdaptiveSta_flg input; VTQD_SpdLim4SetSpd_raw32 input; VTQD_ACCActiveMetSpdHi_raw32 input; VTQD_ACCActiveMetSpdLo_raw32 input; VTQD_Set2MeterSpd_flg input; VTQD_SWC2ScrollUpSta_enum input; VTQD_SWC2ScrollDownSta_enum input; ENUM_SWCBOTTONPRESS_SHORTPRESS parameter; ONE_FLOAT parameter; ENUM_SWCBOTTONPRESS_LONGPRESS parameter; VTQD_ACCSavedSetSpd_raw32 local single; VTQD_SetSpdDeltaLong_raw32 input; VTQD_SetRoadSpdLim_flg input; KTQD_ACCOVRDSpdAdj_flg parameter; KPH2MPH parameter; VTQD_DistanceUnit_flg local boolean; MPH2KPH parameter; KTQD_ACCActiveMetSpdHiMPH_mph parameter; KTQD_ACCActiveMetSpdHi_kph parameter; KTQD_ACCActiveMetSpdLoMPH_mph parameter; KTQD_ACCActiveMetSpdLo_kph parameter; VTQD_RoadSpdActive2Standby_flg local boolean; VINP_Distanceunit_flg input; VTQD_ADASSLIFSpdLimDet_flg input; VTQD_StandbyDisRoadSpd_flg local boolean; VTQD_LScrollPressShort_flg input; FALSE parameter; TRUE parameter; ENUM_SWCBOTTONPRESS_NOPRESS parameter; VVMC_LVDAACCStatusInformation_flg input; VVMC_MeterIndSpeed_raw32 input; VTQD_SWC2ScrollUpSta_flg input; VTQD_SWC2ScrollDownSta_flg input; VTQD_HoldResDet_flg local boolean; VTQD_LastSetSpd_kph input

== stateflow chart tqdtqr_rebuild_V3/Input_Convert/Signal function/Wheel Status Judgment/Whleels State Machine ==
  (default) -> (junction 44)
  (junction 44) -> (junction 46) [order 1] : [VTQD_AllWhlSkip_flg || VINP_DIDGetDynoMode_flg]
      | %add20251014
  (junction 46) -> (junction 48) : {
      | VTQD_WhlSkipSta_enum = ENUM_WHEELSKIPSTA_ALLWHEELS;
      | }
  (junction 44) -> (junction 50) [order 2]
  (junction 50) -> (junction 52) [order 1] : [VTQD_TripleWhlSkip_flg]
  (junction 52) -> (junction 56) [order 1] : [VTQD_RearRFWhlSkip_flg]
  (junction 50) -> (junction 80) [order 2]
  (junction 52) -> (junction 60) [order 2]
  (junction 56) -> (junction 58) : {
      | VTQD_WhlSkipSta_enum = ENUM_WHEELSKIPSTA_REARRF;
      | }
  (junction 60) -> (junction 62) [order 1] : [VTQD_RearLFWhlSkip_flg]
  (junction 60) -> (junction 66) [order 2]
  (junction 62) -> (junction 64) : {
      | VTQD_WhlSkipSta_enum = ENUM_WHEELSKIPSTA_REARLF;
      | }
  (junction 66) -> (junction 68) [order 1] : [VTQD_FrontRRWhlSkip_flg]
  (junction 66) -> (junction 72) [order 2]
  (junction 68) -> (junction 70) : {
      | VTQD_WhlSkipSta_enum = ENUM_WHEELSKIPSTA_FRONTRR;
      | }
  (junction 72) -> (junction 74) [order 1] : [VTQD_FrontLRWhlSkip_flg]
  (junction 72) -> (junction 78) [order 2] : {
      | VTQD_WhlSkipSta_enum = ENUM_WHEELSKIPSTA_STABLE;
      | }
  (junction 74) -> (junction 76) : {
      | VTQD_WhlSkipSta_enum = ENUM_WHEELSKIPSTA_FRONTLR;
      | }
  (junction 82) -> (junction 84) [order 1] : [VTQD_RFLRWhlSkip_flg]
  (junction 80) -> (junction 82) [order 1] : [VTQD_DoubleWhlSkip_flg]
  (junction 82) -> (junction 88) [order 2]
  (junction 84) -> (junction 86) : {
      | VTQD_WhlSkipSta_enum = ENUM_WHEELSKIPSTA_RFLR;
      | }
  (junction 80) -> (junction 120) [order 2]
  (junction 88) -> (junction 90) [order 1] : [VTQD_LFRRWhlSkip_flg]
  (junction 88) -> (junction 94) [order 2]
  (junction 90) -> (junction 92) : {
      | VTQD_WhlSkipSta_enum = ENUM_WHEELSKIPSTA_LFRR;
      | }
  (junction 94) -> (junction 96) [order 1] : [VTQD_RearWhlSkip_flg]
  (junction 94) -> (junction 100) [order 2]
  (junction 96) -> (junction 98) : {
      | VTQD_WhlSkipSta_enum = ENUM_WHEELSKIPSTA_REAR;
      | }
  (junction 100) -> (junction 102) [order 1] : [VTQD_FrontWhlSkip_flg]
  (junction 100) -> (junction 106) [order 2]
  (junction 102) -> (junction 104) : {
      | VTQD_WhlSkipSta_enum = ENUM_WHEELSKIPSTA_FRONT;
      | }
  (junction 106) -> (junction 108) [order 1] : [VTQD_RightWhlSkip_flg]
  (junction 108) -> (junction 110) : {
      | VTQD_WhlSkipSta_enum = ENUM_WHEELSKIPSTA_RIGHT;
      | }
  (junction 106) -> (junction 112) [order 2]
  (junction 112) -> (junction 114) [order 1] : [VTQD_LeftWhlSkip_flg]
  (junction 112) -> (junction 118) [order 2] : {
      | VTQD_WhlSkipSta_enum = ENUM_WHEELSKIPSTA_STABLE;
      | }
  (junction 114) -> (junction 116) : {
      | VTQD_WhlSkipSta_enum = ENUM_WHEELSKIPSTA_LEFT;
      | }
  (junction 120) -> (junction 122) [order 1] : [VTQD_SingleWhlSkip_flg]
  (junction 122) -> (junction 124) [order 1] : [VTQD_RRWhlSkip_flg]
  (junction 120) -> (junction 149) [order 2] : {
      | VTQD_WhlSkipSta_enum = ENUM_WHEELSKIPSTA_STABLE;
      | }
  (junction 122) -> (junction 128) [order 2]
  (junction 124) -> (junction 126) : {
      | VTQD_WhlSkipSta_enum = ENUM_WHEELSKIPSTA_RR;
      | }
  (junction 128) -> (junction 130) [order 1] : [VTQD_LRWhlSkip_flg]
  (junction 128) -> (junction 134) [order 2]
  (junction 130) -> (junction 132) : {
      | VTQD_WhlSkipSta_enum = ENUM_WHEELSKIPSTA_LR;
      | }
  (junction 134) -> (junction 136) [order 1] : [VTQD_RFWhlSkip_flg]
  (junction 134) -> (junction 141) [order 2]
  (junction 136) -> (junction 138) : {
      | VTQD_WhlSkipSta_enum = ENUM_WHEELSKIPSTA_RF;
      | }
  (junction 141) -> (junction 143) [order 1] : [VTQD_LFWhlSkip_flg]
  (junction 141) -> (junction 147) [order 2] : {
      | VTQD_WhlSkipSta_enum = ENUM_WHEELSKIPSTA_STABLE;
      | }
  (junction 143) -> (junction 145) : {
      | VTQD_WhlSkipSta_enum = ENUM_WHEELSKIPSTA_LF;
      | }
  data: ENUM_WHEELSKIPSTA_STABLE parameter; ENUM_WHEELSKIPSTA_LF parameter; ENUM_WHEELSKIPSTA_RF parameter; ENUM_WHEELSKIPSTA_LR parameter; ENUM_WHEELSKIPSTA_RR parameter; ENUM_WHEELSKIPSTA_LEFT parameter; ENUM_WHEELSKIPSTA_RIGHT parameter; ENUM_WHEELSKIPSTA_FRONT parameter; ENUM_WHEELSKIPSTA_REAR parameter; ENUM_WHEELSKIPSTA_LFRR parameter; ENUM_WHEELSKIPSTA_RFLR parameter; ENUM_WHEELSKIPSTA_FRONTLR parameter; ENUM_WHEELSKIPSTA_FRONTRR parameter; ENUM_WHEELSKIPSTA_REARLF parameter; ENUM_WHEELSKIPSTA_REARRF parameter; ENUM_WHEELSKIPSTA_ALLWHEELS parameter; VTQD_LFWhlSkip_flg input; VTQD_RFWhlSkip_flg input; VTQD_LRWhlSkip_flg input; VTQD_RRWhlSkip_flg input; VTQD_SingleWhlSkip_flg input; VTQD_LeftWhlSkip_flg input; VTQD_RightWhlSkip_flg input; VTQD_FrontWhlSkip_flg input; VTQD_RearWhlSkip_flg input; VTQD_LFRRWhlSkip_flg input; VTQD_RFLRWhlSkip_flg input; VTQD_DoubleWhlSkip_flg input; VTQD_FrontLRWhlSkip_flg input; VTQD_FrontRRWhlSkip_flg input; VTQD_RearLFWhlSkip_flg input; VTQD_RearRFWhlSkip_flg input; VTQD_TripleWhlSkip_flg input; VTQD_AllWhlSkip_flg input; VTQD_WhlSkipSta_enum output uint8; VINP_DIDGetDynoMode_flg input
